simulink model "array_sum"  (R2013b)
settings: Solver=ode45  StartTime=0.0  StopTime=10.0  RelTol=1e-3
settings Model: Creator=Chris  LastModifiedBy=Chris

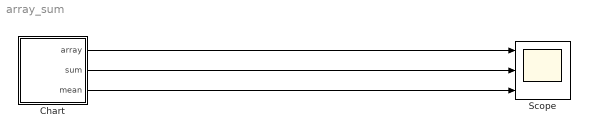
== system array_sum ==
  Chart : Stateflow chart  TreatAsAtomicUnit=on
  Scope : Scope  NumInputPorts=3
      settings: YMin=1~0~-5  YMax=3~7.5~5
  wires:
  Chart/2(sum) -> Scope/2
  Chart/1(array) -> Scope/1
  Chart/3(mean) -> Scope/3

== stateflow chart array_sum/Chart ==
  state init
    array[0] = 1;
    array[1] = 2;
    array[2] = 3;
    array[3] = 4;
    array[4] = 5;
    array[5] = 6;
    array[6] = 7;
    array[7] = 8;
    length = 8;
    sum = 0;
  state Sum_and_Mean
    (junction 6) -> (junction 4) [order 1] : [i < length]
    (junction 4) -> (junction 5) : {sum = sum + array[i];}
    (junction 7) -> (junction 6) : {i = 0;}
    (junction 5) -> (junction 6) : {i = i + 1;}
    (junction 6) -> (junction 3) [order 2]
    (junction 3) -> (junction 31) : {mean = sum / length;}
  state Done
  init -> (junction 7)
  (default) -> init
  (junction 31) -> Done
  data: array output double size=8; i local double; sum output double; mean output double; length local double
